simulink model "Exercise_3_Simulink"  (R2024b)
settings: Solver=VariableStepAuto  StartTime=0.0  StopTime=4*pi/(8+1)  RelTol=1e-3
undefined symbols (not defined in the file): alpha, k_1, k_2, r, x_i, y_i, zeta
libraries: simulink x8, robotmobilelib x2
settings Model: Creator=monet  LastModifiedBy=monet

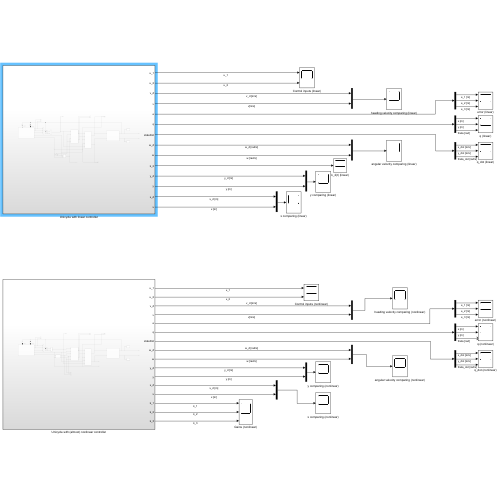
[thumbnail: Simulink's stored preview of the top-level diagram]
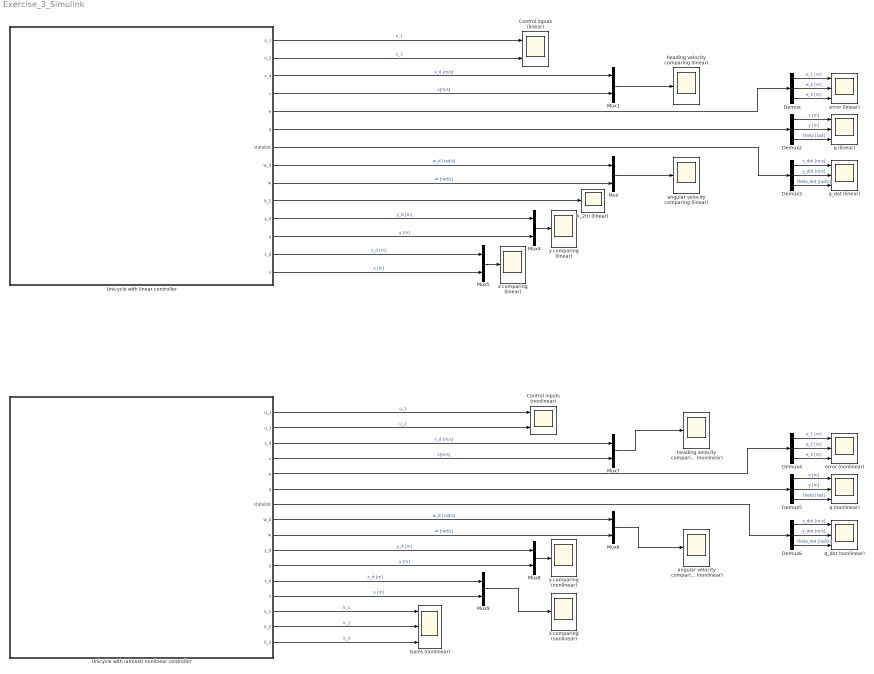
== system Exercise_3_Simulink ==
  Control inputs (linear) : Scope  NumInputPorts=2
  Control inputs (nonlinear) : Scope  NumInputPorts=2
  Demux{,2..6} (6 alike) : Demux  Outputs=3
  Gains (nonlinear) : Scope  NumInputPorts=3
  Mux{,1,4..9} (8 alike) : Mux  Inputs=2
  Unicycle with (almost) nonlinear controller : Subsystem
  Unicycle with linear controller : Subsystem
  angular velocity comparing (linear) : Scope
  angular velocity comparing (nonlinear) : Scope
  error (linear) : Scope  NumInputPorts=3
  error (nonlinear) : Scope  NumInputPorts=3
  heading velocity comparing (linear) : Scope
  heading velocity comparing (nonlinear) : Scope
  k_2(t) (linear) : Scope
  q (linear) : Scope  NumInputPorts=3
  q (nonlinear) : Scope  NumInputPorts=3
  q_dot (linear) : Scope  NumInputPorts=3
  q_dot (nonlinear) : Scope  NumInputPorts=3
  x comparing (linear) : Scope
  x comparing (nonlinear) : Scope
  y comparing (linear) : Scope
  y comparing (nonlinear) : Scope
  wires:
  Mux/1 -> angular velocity comparing (linear)/1
  Unicycle with linear controller/1(u_1) -> Control inputs (linear)/1  "u_1"
  Unicycle with linear controller/3(v_d) -> Mux1/1  "v_d [m/s]"
  Unicycle with linear controller/5(e) -> Demux/1
  Unicycle with linear controller/4(v) -> Mux1/2  "v[m/s]"
  Unicycle with linear controller/2(u_2) -> Control inputs (linear)/2  "u_2"
  Unicycle with linear controller/6(q) -> Demux2/1
  Unicycle with linear controller/7(stateDot) -> Demux3/1
  Unicycle with linear controller/8(w_d) -> Mux/1  "w_d [rad/s]"
  Unicycle with linear controller/10(k_2) -> k_2(t) (linear)/1
  Unicycle with linear controller/9(w) -> Mux/2  "w [rad/s]"
  Unicycle with linear controller/11(y_d) -> Mux4/1  "y_d [m]"
  Unicycle with linear controller/12(y) -> Mux4/2  "y [m]"
  Unicycle with linear controller/13(x_d) -> Mux5/1  "x_d [m]"
  Unicycle with linear controller/14(x) -> Mux5/2  "x [m]"
  Unicycle with (almost) nonlinear controller/6(q) -> Demux5/1
  Unicycle with (almost) nonlinear controller/7(stateDot) -> Demux6/1
  Unicycle with (almost) nonlinear controller/2(u_2) -> Control inputs (nonlinear)/2  "u_2"
  Unicycle with (almost) nonlinear controller/5(e) -> Demux4/1
  Unicycle with (almost) nonlinear controller/1(u_1) -> Control inputs (nonlinear)/1  "u_1"
  Unicycle with (almost) nonlinear controller/14(k_1) -> Gains (nonlinear)/1  "k_1"
  Unicycle with (almost) nonlinear controller/15(k_2) -> Gains (nonlinear)/2  "k_2"
  Unicycle with (almost) nonlinear controller/16(k_3) -> Gains (nonlinear)/3  "k_3"
  Demux/1 -> error (linear)/1  "e_1 [m]"
  Demux/2 -> error (linear)/2  "e_2 [m]"
  Demux/3 -> error (linear)/3  "e_3 [m]"
  Demux2/2 -> q (linear)/2  "y [m]"
  Demux2/1 -> q (linear)/1  "x [m]"
  Demux2/3 -> q (linear)/3  "theta [rad]"
  Demux3/2 -> q_dot (linear)/2  "y_dot [m/s]"
  Demux3/1 -> q_dot (linear)/1  "x_dot [m/s]"
  Demux3/3 -> q_dot (linear)/3  "theta_dot [rad/s]"
  Demux6/1 -> q_dot (nonlinear)/1  "x_dot [m/s]"
  Demux6/2 -> q_dot (nonlinear)/2  "y_dot [m/s]"
  Demux4/3 -> error (nonlinear)/3  "e_3 [m]"
  Demux4/1 -> error (nonlinear)/1  "e_1 [m]"
  Demux4/2 -> error (nonlinear)/2  "e_2 [m]"
  Demux5/1 -> q (nonlinear)/1  "x [m]"
  Demux5/3 -> q (nonlinear)/3  "theta [rad]"
  Demux5/2 -> q (nonlinear)/2  "y [m]"
  Demux6/3 -> q_dot (nonlinear)/3  "theta_dot [rad/s]"
  Mux1/1 -> heading velocity comparing (linear)/1
  Mux4/1 -> y comparing (linear)/1
  Mux5/1 -> x comparing (linear)/1
  Mux9/1 -> x comparing (nonlinear)/1
  Mux6/1 -> angular velocity comparing (nonlinear)/1
  Mux7/1 -> heading velocity comparing (nonlinear)/1
  Unicycle with (almost) nonlinear controller/13(x) -> Mux9/2  "x [m]"
  Unicycle with (almost) nonlinear controller/4(v) -> Mux7/2  "v[m/s]"
  Unicycle with (almost) nonlinear controller/12(x_d) -> Mux9/1  "x_d [m]"
  Mux8/1 -> y comparing (nonlinear)/1
  Unicycle with (almost) nonlinear controller/11(y) -> Mux8/2  "y [m]"
  Unicycle with (almost) nonlinear controller/10(y_d) -> Mux8/1  "y_d [m]"
  Unicycle with (almost) nonlinear controller/3(v_d) -> Mux7/1  "v_d [m/s]"
  Unicycle with (almost) nonlinear controller/8(w_d) -> Mux6/1  "w_d [rad/s]"
  Unicycle with (almost) nonlinear controller/9(w) -> Mux6/2  "w [rad/s]"

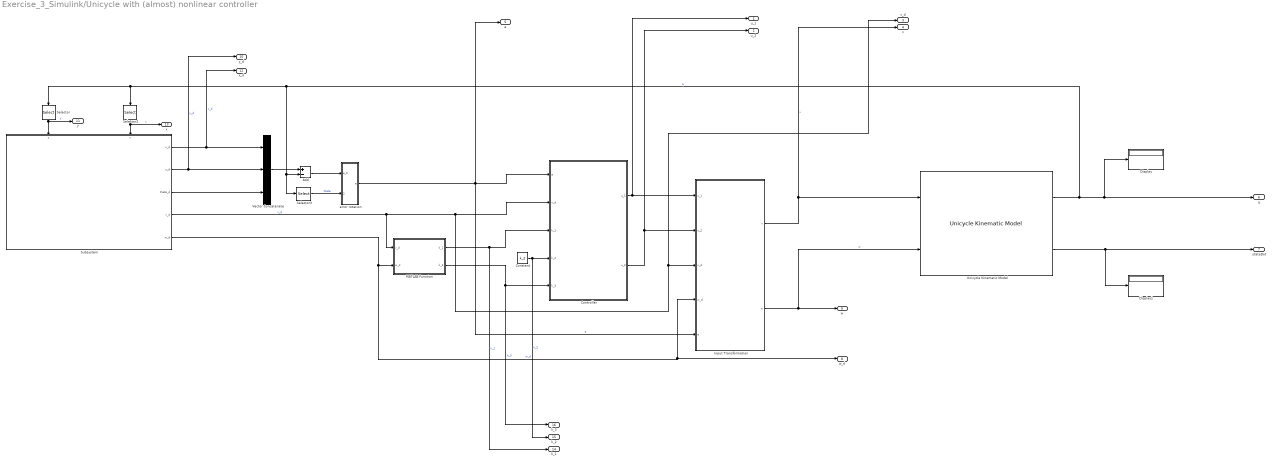
== system Exercise_3_Simulink/Unicycle with (almost) nonlinear controller ==
  Add : Sum  Inputs=+-
  Constant : Constant  Value=k_2
  Controller : MATLAB Function  TreatAsAtomicUnit=on
  Display : Display
  Display1 : Display
  Input Transformation : MATLAB Function  TreatAsAtomicUnit=on
  MATLAB Function : MATLAB Function  TreatAsAtomicUnit=on
  Selector : Selector  InputPortWidth=3  IndexOptions=Index vector (dialog)  Indices=2  OutputSizes=1  RuntimeRangeChecks=on
  Selector2 : Selector  InputPortWidth=3  IndexOptions=Index vector (dialog)  Indices=[1]  OutputSizes=1  RuntimeRangeChecks=on
  Selector3 : Selector  InputPortWidth=3  IndexOptions=Index vector (dialog)  Indices=3  OutputSizes=1
  Subsystem : Subsystem
      settings: PortSchema="{\"entries\":[{\"content\":{\"sides\":[{\"content\":{},\"type\":\"ConnectorPlacement.EquallySpacedRectSide\",\"uuid\":\"5e1ef72e-e14b-4fc5-86a2-e7b300b76291\"},{\"content\":{\"connectorIds\":[\"Out1\",\"Out2\",\"Out3\",\"Out4\",\"Out5\"],\"side\":\"RIGHT\"},\"type\":\"ConnectorPlacement.EquallySpacedRectSide\",\"uuid\":\"f3f998ca-b69f-453a-813f-7c460b5f2423\"},{\"content\":{\"connectorIds\":[\"In1\",\"In2\"],\"side\":\"TOP\"},\"type\":\"ConnectorPlacement.EquallySpacedRectSide\",\"uuid\":\"f96d88d6-9967-4a2e-bba2-c83fe34b21ff\"}]},\"type\":\"ConnectorPlacement.EquallySpacedConnector\",\"uuid\":\"8a367af1-f6a3-4926-804f-000103b3b3fa\"}],\"packageUris\":[\"http://schema.mathworks.com/mf0/Connector/R2020b\"],\"version\":\"1.0\"}"
  Unicycle Kinematic Model : robotmobilelib/Unicycle Kinematic Model  VehicleInputs=Vehicle Speed & Heading Angular Velocity  WheelRadius=0.1  WheelSpeedRange=[-Inf Inf]  InitialState=[x_i; y_i; 0]  SimulateUsing=Interpreted execution
  Vector Concatenate : Concatenate  NumInputs=3
  error rotation : MATLAB Function  TreatAsAtomicUnit=on
  u_1 : Outport
  u_2 : Outport  Port=2
  v_d : Outport  Port=3
  v : Outport  Port=4
  e : Outport  Port=5
  q : Outport  Port=6
  stateDot : Outport  Port=7
  w_d : Outport  Port=8
  w : Outport  Port=9
  y_d : Outport  Port=10
  y : Outport  Port=11
  x_d : Outport  Port=12
  x : Outport  Port=13
  k_1 : Outport  Port=14
  k_2 : Outport  Port=15
  k_3 : Outport  Port=16
  wires:
  Subsystem/5(w_d) -> MATLAB Function/2(w_d), w_d/1, Input Transformation/4(w_d)  "w_d"
  Subsystem/4(v_d) -> MATLAB Function/1(v_d), Controller/2(v_d), Input Transformation/3(v_d), v_d/1  "v_d"
  Input Transformation/2(w) -> w/1, Unicycle Kinematic Model/2  "w"
  Subsystem/2(y_d) -> y_d/1, Vector Concatenate/2  "y_d"
  Subsystem/1(x_d) -> Vector Concatenate/1, x_d/1  "x_d"
  Unicycle Kinematic Model/1 -> Selector3/1, Add/2, Selector/1, Selector2/1, q/1, Display/1  "q"
  Selector2/1 -> x/1, Subsystem/2(x)  "x"
  error rotation/1(e) -> e/1, Controller/1(e), Input Transformation/5(e)  "e"
  Controller/2(u_2) -> u_2/1, Input Transformation/2(u_2)
  Selector3/1 -> error rotation/2(theta)  "theta"
  Controller/1(u_1) -> u_1/1, Input Transformation/1(u_1)
  Input Transformation/1(v) -> v/1, Unicycle Kinematic Model/1  "v"
  Vector Concatenate/1 -> Add/1
  Subsystem/3(theta_d) -> Vector Concatenate/3
  Unicycle Kinematic Model/2 -> stateDot/1, Display1/1
  Add/1 -> error rotation/1(e_0)
  Selector/1 -> Subsystem/1(y), y/1  "y"
  Constant/1 -> Controller/4(k_2), k_2/1  "k_2"
  MATLAB Function/1(k_1) -> k_1/1, Controller/3(k_1)  "k_1"
  MATLAB Function/2(k_3) -> k_3/1, Controller/5(k_3)  "k_3"

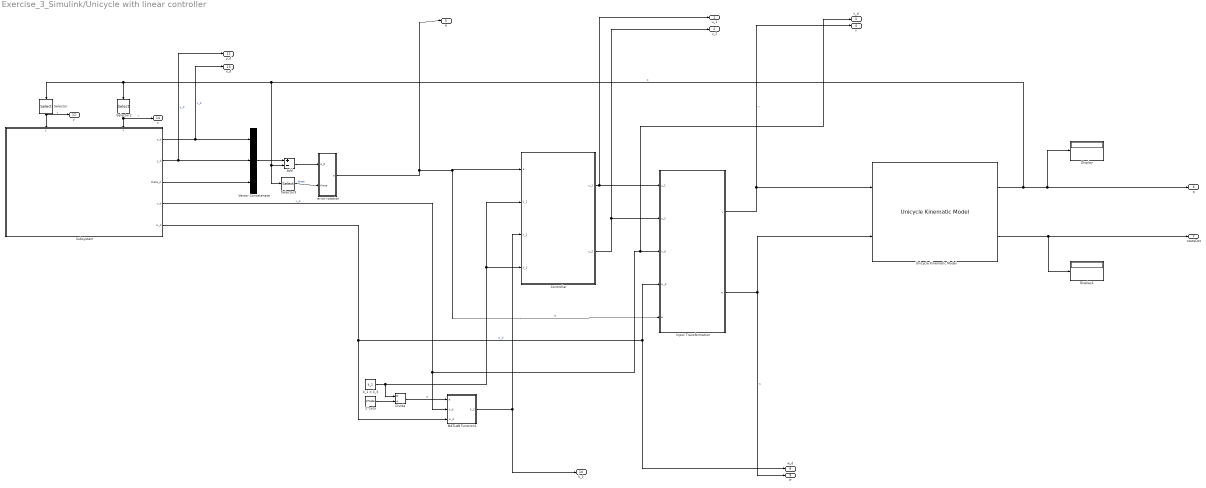
== system Exercise_3_Simulink/Unicycle with linear controller ==
  2*zeta : Constant  Value=2*zeta
  Add : Sum  Inputs=+-
  Controller : MATLAB Function  TreatAsAtomicUnit=on
  Display : Display
  Display1 : Display
  Divide : Product  Inputs=*/
  Input Transformation : MATLAB Function  TreatAsAtomicUnit=on
  MATLAB Function1 : MATLAB Function  TreatAsAtomicUnit=on
  Selector : Selector  InputPortWidth=3  IndexOptions=Index vector (dialog)  Indices=2  OutputSizes=1  RuntimeRangeChecks=on
  Selector2 : Selector  InputPortWidth=3  IndexOptions=Index vector (dialog)  Indices=[1]  OutputSizes=1  RuntimeRangeChecks=on
  Selector3 : Selector  InputPortWidth=3  IndexOptions=Index vector (dialog)  Indices=3  OutputSizes=1
  Subsystem : Subsystem
      settings: PortSchema="{\"entries\":[{\"content\":{\"sides\":[{\"content\":{},\"type\":\"ConnectorPlacement.EquallySpacedRectSide\",\"uuid\":\"5e1ef72e-e14b-4fc5-86a2-e7b300b76291\"},{\"content\":{\"connectorIds\":[\"Out1\",\"Out2\",\"Out3\",\"Out4\",\"Out5\"],\"side\":\"RIGHT\"},\"type\":\"ConnectorPlacement.EquallySpacedRectSide\",\"uuid\":\"f3f998ca-b69f-453a-813f-7c460b5f2423\"},{\"content\":{\"connectorIds\":[\"In1\",\"In2\"],\"side\":\"TOP\"},\"type\":\"ConnectorPlacement.EquallySpacedRectSide\",\"uuid\":\"f96d88d6-9967-4a2e-bba2-c83fe34b21ff\"}]},\"type\":\"ConnectorPlacement.EquallySpacedConnector\",\"uuid\":\"8a367af1-f6a3-4926-804f-000103b3b3fa\"}],\"packageUris\":[\"http://schema.mathworks.com/mf0/Connector/R2020b\"],\"version\":\"1.0\"}"
  Unicycle Kinematic Model : robotmobilelib/Unicycle Kinematic Model  VehicleInputs=Vehicle Speed & Heading Angular Velocity  WheelRadius=0.1  WheelSpeedRange=[-Inf Inf]  InitialState=[x_i; y_i; 0]  SimulateUsing=Interpreted execution
  Vector Concatenate : Concatenate  NumInputs=3
  error rotation : MATLAB Function  TreatAsAtomicUnit=on
  k_1 = k_3 : Constant  Value=k_1
  u_1 : Outport
  u_2 : Outport  Port=2
  v_d : Outport  Port=3
  v : Outport  Port=4
  e : Outport  Port=5
  q : Outport  Port=6
  stateDot : Outport  Port=7
  w_d : Outport  Port=8
  w : Outport  Port=9
  k_2 : Outport  Port=10
  y_d : Outport  Port=11
  y : Outport  Port=12
  x_d : Outport  Port=13
  x : Outport  Port=14
  wires:
  Subsystem/5(w_d) -> w_d/1, Input Transformation/4(w_d), MATLAB Function1/3(w_d)  "w_d"
  Subsystem/4(v_d) -> MATLAB Function1/2(v_d), v_d/1, Input Transformation/3(v_d)  "v_d"
  Input Transformation/2(w) -> w/1, Unicycle Kinematic Model/2  "w"
  2*zeta/1 -> Divide/2
  Subsystem/2(y_d) -> y_d/1, Vector Concatenate/2  "y_d"
  Subsystem/1(x_d) -> Vector Concatenate/1, x_d/1  "x_d"
  Unicycle Kinematic Model/1 -> Selector3/1, Add/2, Selector/1, Selector2/1, q/1, Display/1  "q"
  Selector2/1 -> x/1, Subsystem/2(x)  "x"
  error rotation/1(e) -> e/1, Input Transformation/5(e), Controller/1(e)  "e"
  Controller/2(u_2) -> u_2/1, Input Transformation/2(u_2)
  Selector3/1 -> error rotation/2(theta)  "theta"
  Controller/1(u_1) -> u_1/1, Input Transformation/1(u_1)
  Input Transformation/1(v) -> v/1, Unicycle Kinematic Model/1  "v"
  Vector Concatenate/1 -> Add/1
  Subsystem/3(theta_d) -> Vector Concatenate/3
  Divide/1 -> MATLAB Function1/1(a)  "a"
  Unicycle Kinematic Model/2 -> stateDot/1, Display1/1
  MATLAB Function1/1(k_2) -> k_2/1, Controller/3(k_2)
  k_1 = k_3/1 -> Controller/2(k_1), Controller/4(k_3), Divide/1
  Add/1 -> error rotation/1(e_0)
  Selector/1 -> Subsystem/1(y), y/1  "y"

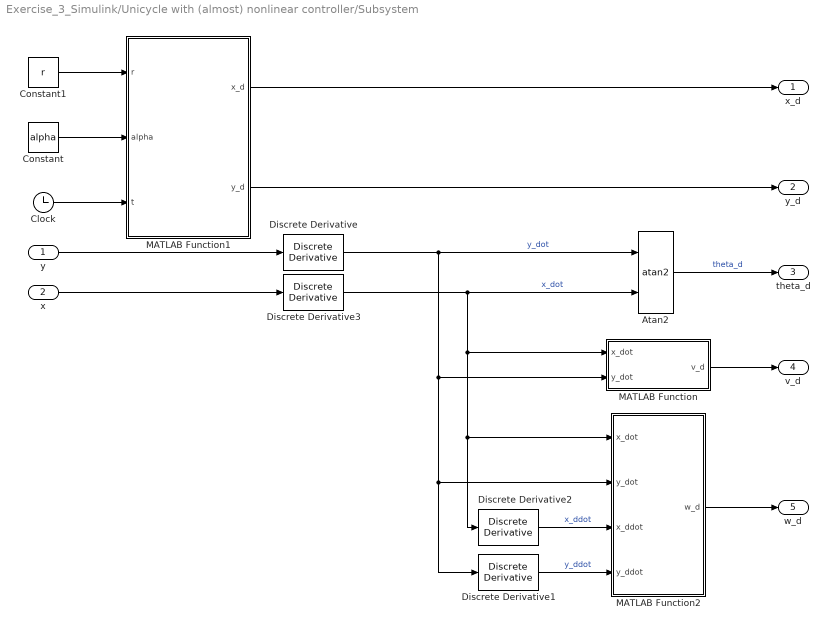
== system Exercise_3_Simulink/Unicycle with (almost) nonlinear controller/Subsystem ==
  y : Inport
  x : Inport  Port=2
  Atan2 : Trigonometry  Operator=atan2
  Clock : Clock
  Constant : Constant  Value=alpha
  Constant1 : Constant  Value=r
  Discrete Derivative{,1..3} (4 alike) : simulink/Quick Insert/Discrete/Discrete Derivative  gainval=1.0  ICPrevScaledInput=0.0  OutMin=[]  OutMax=[]  OutDataType=fixdt(1, 16)  OutScaling=2^-10  DoSatur=off
  MATLAB Function : MATLAB Function  TreatAsAtomicUnit=on
  MATLAB Function1 : MATLAB Function  TreatAsAtomicUnit=on
  MATLAB Function2 : MATLAB Function  TreatAsAtomicUnit=on
  x_d : Outport
  y_d : Outport  Port=2
  theta_d : Outport  Port=3
  v_d : Outport  Port=4
  w_d : Outport  Port=5
  wires:
  Constant1/1 -> MATLAB Function1/1(r)
  MATLAB Function1/2(y_d) -> y_d/1
  Discrete Derivative3/1 -> Discrete Derivative2/1, MATLAB Function2/1(x_dot), MATLAB Function/1(x_dot), Atan2/2  "x_dot"
  MATLAB Function1/1(x_d) -> x_d/1
  Constant/1 -> MATLAB Function1/2(alpha)
  Clock/1 -> MATLAB Function1/3(t)
  Atan2/1 -> theta_d/1  "theta_d"
  MATLAB Function/1(v_d) -> v_d/1
  MATLAB Function2/1(w_d) -> w_d/1
  Discrete Derivative/1 -> Discrete Derivative1/1, MATLAB Function2/2(y_dot), MATLAB Function/2(y_dot), Atan2/1  "y_dot"
  Discrete Derivative2/1 -> MATLAB Function2/3(x_ddot)  "x_ddot"
  Discrete Derivative1/1 -> MATLAB Function2/4(y_ddot)  "y_ddot"
  x/1 -> Discrete Derivative3/1
  y/1 -> Discrete Derivative/1

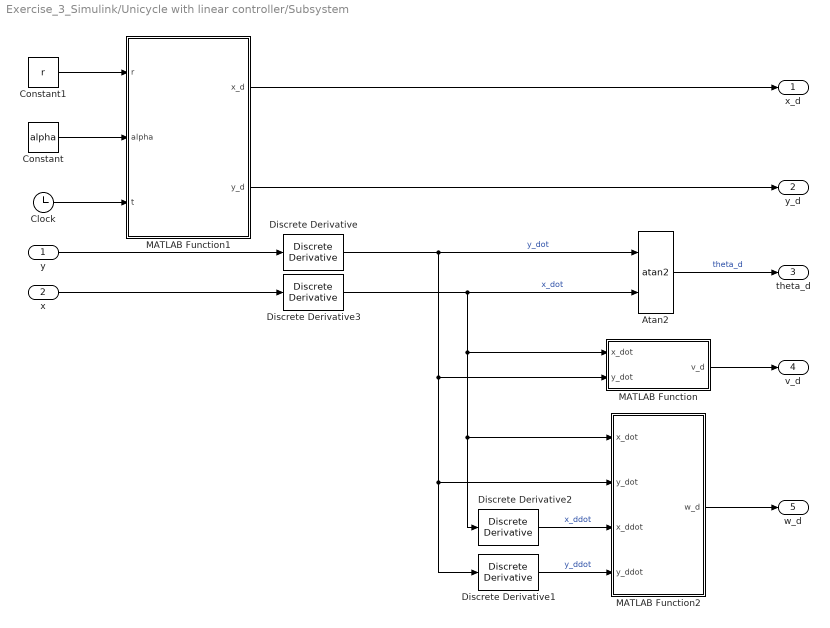
== system Exercise_3_Simulink/Unicycle with linear controller/Subsystem ==
  y : Inport
  x : Inport  Port=2
  Atan2 : Trigonometry  Operator=atan2
  Clock : Clock
  Constant : Constant  Value=alpha
  Constant1 : Constant  Value=r
  Discrete Derivative{,1..3} (4 alike) : simulink/Quick Insert/Discrete/Discrete Derivative  gainval=1.0  ICPrevScaledInput=0.0  OutMin=[]  OutMax=[]  OutDataType=fixdt(1, 16)  OutScaling=2^-10  DoSatur=off
  MATLAB Function : MATLAB Function  TreatAsAtomicUnit=on
  MATLAB Function1 : MATLAB Function  TreatAsAtomicUnit=on
  MATLAB Function2 : MATLAB Function  TreatAsAtomicUnit=on
  x_d : Outport
  y_d : Outport  Port=2
  theta_d : Outport  Port=3
  v_d : Outport  Port=4
  w_d : Outport  Port=5
  wires:
  Constant1/1 -> MATLAB Function1/1(r)
  MATLAB Function1/2(y_d) -> y_d/1
  Discrete Derivative3/1 -> Discrete Derivative2/1, MATLAB Function2/1(x_dot), MATLAB Function/1(x_dot), Atan2/2  "x_dot"
  MATLAB Function1/1(x_d) -> x_d/1
  Constant/1 -> MATLAB Function1/2(alpha)
  Clock/1 -> MATLAB Function1/3(t)
  Atan2/1 -> theta_d/1  "theta_d"
  MATLAB Function/1(v_d) -> v_d/1
  MATLAB Function2/1(w_d) -> w_d/1
  Discrete Derivative/1 -> Discrete Derivative1/1, MATLAB Function2/2(y_dot), MATLAB Function/2(y_dot), Atan2/1  "y_dot"
  Discrete Derivative2/1 -> MATLAB Function2/3(x_ddot)  "x_ddot"
  Discrete Derivative1/1 -> MATLAB Function2/4(y_ddot)  "y_ddot"
  x/1 -> Discrete Derivative3/1
  y/1 -> Discrete Derivative/1

== matlab function Exercise_3_Simulink/Unicycle with (almost) nonlinear controller/MATLAB Function ==
  data: v_d input; k_1 output; w_d input; k_3 output
function [k_1,k_3] = fcn(v_d,w_d)

k_1 = 1+v_d^2,2;
k_3 = norm(v_d^2/15+w_d^2/100,2);

end

== matlab function Exercise_3_Simulink/Unicycle with (almost) nonlinear controller/Subsystem/MATLAB Function ==
  data: x_dot input; v_d output; y_dot input
function v_d = fcn(x_dot,y_dot)
    v_d = sqrt(x_dot^2 + y_dot^2);
end

== matlab function Exercise_3_Simulink/Unicycle with (almost) nonlinear controller/Subsystem/MATLAB Function1 ==
  data: r input; x_d output; alpha input; t input; y_d output
function [x_d,y_d] = fcn(r,alpha,t)
    x_d = r*cos((alpha+1)*t)/(1+(sin((alpha+1)*t)^2));
    y_d = r*cos((alpha+1)*t)*sin((alpha+1)*t)./(1+(sin((alpha+1)*t)^2));
end

== matlab function Exercise_3_Simulink/Unicycle with (almost) nonlinear controller/Subsystem/MATLAB Function2 ==
  data: x_dot input; w_d output; y_dot input; x_ddot input; y_ddot input
function w_d = fcn(x_dot,y_dot,x_ddot,y_ddot)
    w_d = (y_ddot*x_dot - x_ddot*y_dot)/(x_dot^2 + y_dot^2);
end

== matlab function Exercise_3_Simulink/Unicycle with linear controller/Subsystem/MATLAB Function1 ==
  data: r input; x_d output; alpha input; t input; y_d output
function [x_d,y_d] = fcn(r,alpha,t)
    x_d = r*cos((alpha+1)*t)/(1+(sin((alpha+1)*t)^2));
    y_d = r*cos((alpha+1)*t)*sin((alpha+1)*t)./(1+(sin((alpha+1)*t)^2));
end

== matlab function Exercise_3_Simulink/Unicycle with (almost) nonlinear controller/error rotation ==
  data: e_0 input; e output; theta input
function e  = fcn(e_0,theta)
M = [cos(theta) sin(theta) 0;
    -sin(theta) cos(theta) 0;
    0 0 1];
e = M*e_0;
end

== matlab function Exercise_3_Simulink/Unicycle with linear controller/Controller ==
  data: e input; u_1 output; u_2 output; k_1 input; k_2 input; k_3 input

function [u_1,u_2] = fcn(e,k_1,k_2,k_3)
    u_1 = -k_1*e(1,1);
    u_2 = -k_2*e(2,1) - k_3*e(3,1);
end

== matlab function Exercise_3_Simulink/Unicycle with linear controller/Subsystem/MATLAB Function ==
  data: x_dot input; v_d output; y_dot input
function v_d = fcn(x_dot,y_dot)
    v_d = sqrt(x_dot^2 + y_dot^2);
end

== matlab function Exercise_3_Simulink/Unicycle with linear controller/Subsystem/MATLAB Function2 ==
  data: x_dot input; w_d output; y_dot input; x_ddot input; y_ddot input
function w_d = fcn(x_dot,y_dot,x_ddot,y_ddot)
    w_d = (y_ddot*x_dot - x_ddot*y_dot)/(x_dot^2 + y_dot^2);
end

== matlab function Exercise_3_Simulink/Unicycle with linear controller/MATLAB Function1 ==
  data: a input; v_d input; k_2 output; w_d input
function k_2 = fcn(a,v_d,w_d)
    k_2 = (a^2-w_d)/v_d;
end

== matlab function Exercise_3_Simulink/Unicycle with linear controller/Input Transformation ==
  data: u_1 input; v output; u_2 input; v_d input; w_d input; e input; w output
function [v,w] = fcn(u_1,u_2,v_d,w_d,e)
v = v_d*cos(e(3,1)) - u_1;
w = w_d - u_2;
end

== matlab function Exercise_3_Simulink/Unicycle with linear controller/error rotation ==
  data: e_0 input; e output; theta input
function e  = fcn(e_0,theta)
M = [cos(theta) sin(theta) 0;
    -sin(theta) cos(theta) 0;
    0 0 1];
e = M*e_0;
end

== matlab function Exercise_3_Simulink/Unicycle with (almost) nonlinear controller/Controller ==
  data: e input; v_d input; u_1 output; u_2 output; k_1 input; k_2 input; k_3 input

function [u_1,u_2] = fcn(e,v_d,k_1,k_2,k_3)
    u_1 = -k_1*e(1,1);
    u_2 = -k_2*v_d*sinc(e(3,1))*e(2,1) - k_3*e(3,1);
end

== matlab function Exercise_3_Simulink/Unicycle with (almost) nonlinear controller/Input Transformation ==
  data: u_1 input; v output; u_2 input; v_d input; w_d input; e input; w output
function [v,w] = fcn(u_1,u_2,v_d,w_d,e)
v = v_d*cos(e(3,1)) - u_1;
w = w_d - u_2;
end
